simulink model "Microgrid"  (R2022b)
settings: Solver=ode45  StartTime=0.0  StopTime=0.5  RelTol=1e-3  EnableMultiTasking=on
undefined symbols (not defined in the file): AFPV, AFW, BMSS1, c1, c2, c3, c4, c5, c6, D1, Delta, DG, Ion, Lithium, pvc, R, wf1
libraries: spsDiodeLib x10, spsVoltageMeasurementLib x8, spsThreePhaseVIMeasurementLib x7, spsSeriesRLCBranchLib x7, fuzblock x6, sps_avr x5, spsMosfetLib x3, powerlib_extras x3, spsBreakerLib x2, spsThreePhaseParallelRLCLoadLib x2, spsThreePhaseBreakerLib x2, spsPWMGenerator2LevelLib x2
(part 1 of 2)
settings Model: Creator=Indhu  LastModifiedBy=zs
settings SolverCC: AlgebraicLoopSolver=TrustRegion
settings DataIOCC: LimitDataPoints=on  SaveFormat=Array  ReturnWorkspaceOutputs=off
settings OptimizationCC: LifeSpan=inf
settings DebuggingCC: SolverPrmCheckMsg=warning  UnconnectedInputMsg=warning  UnconnectedOutputMsg=warning  UnconnectedLineMsg=warning  SFUnexpectedBacktrackingDiag=warning  SFNoUnconditionalDefaultTransitionDiag=warning  SFExecutionAtInitializationDiag=none  SFMachineParentedDataDiag=warning  ArithmeticOperatorsInVariantConditions=warning
settings HardwareCC: ProdBitPerPointer=32  ProdBitPerSizeT=32  ProdBitPerPtrDiffT=32  ProdLargestAtomicFloat=None  ProdIntDivRoundTo=Undefined  ProdEndianess=Unspecified  ProdWordSize=32  ProdHWDeviceType=32-bit Generic
settings ModelReferenceCC: EnableRefExpFcnMdlSchedulingChecks=on  PropagateSignalLabelsOutOfModel=off
settings SFSimCC: SimUseLocalCustomCode=off  CustomCodeUndefinedFunction=UseInterfaceOnly
settings RTWCC: RTWUseLocalCustomCode=off
settings CodeAppCC: StateflowObjectComments=on
settings GRTTargetCC: TargetLangStandard=C89/C90 (ANSI)
settings ConfigComp: CovMetricSettings=dw  CovSaveCumulativeToWorkspaceVar=on  CovSaveSingleToWorkspaceVar=on  CovExternalEMLEnable=off  CovSFcnEnable=off
settings SimscapeCC: SimscapeNormalizeSystem=off

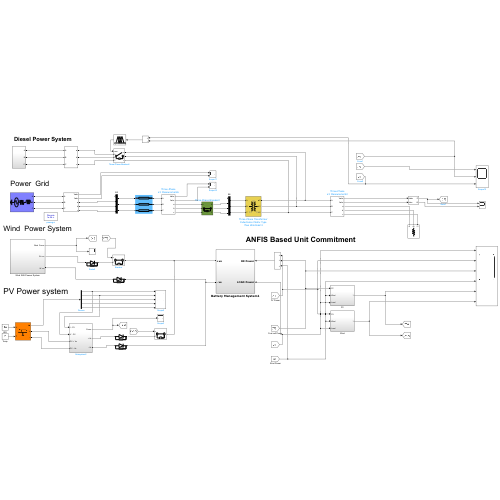
[thumbnail: Simulink's stored preview of the top-level diagram]
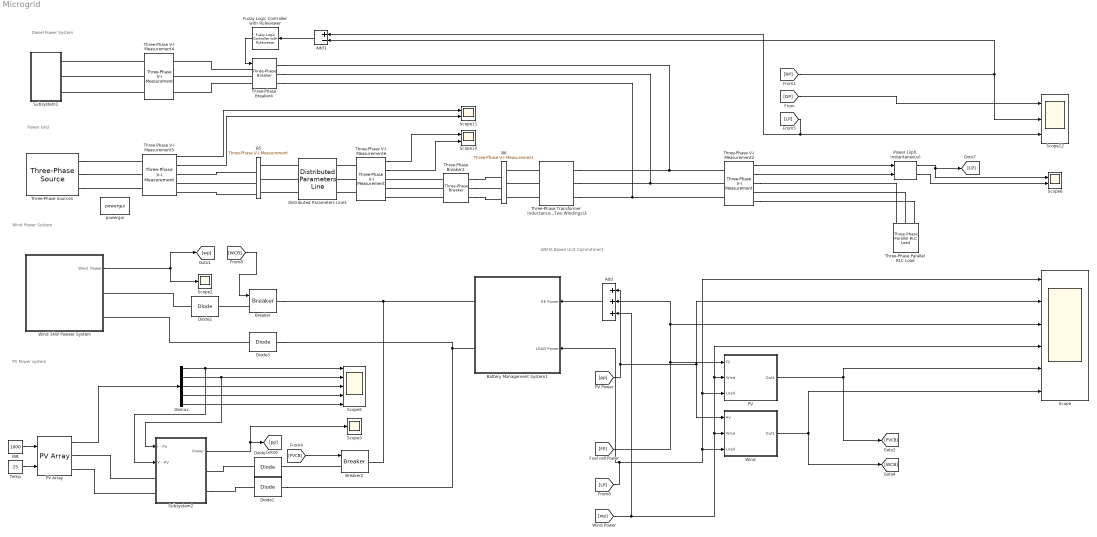
== system Microgrid ==
  note: ANFIS Based Unit Commitment
  note: Power Grid
  note: Wind Power System
  note: PV Power system
  note: Diesel Power System
  Add : Sum  Inputs=+++
  Add1 : Sum  Inputs=+-
  B5 : spsThreePhaseVIMeasurementLib/Three-Phase V-I Measurement  VoltageMeasurement=phase-to-ground  SetLabelV=off  LabelV=Vabc_B12  Vpu=off  VpuLL=off  CurrentMeasurement=no  SetLabelI=off  LabelI=A1  Ipu=off  Pbase=100e6  Vbase=25e3  OutputType=Magnitude  PhasorSimulation=off  PSBequivalent=0
  B6 : spsThreePhaseVIMeasurementLib/Three-Phase V-I Measurement  VoltageMeasurement=phase-to-phase  SetLabelV=off  LabelV=Vabc_B12  Vpu=off  VpuLL=off  CurrentMeasurement=no  SetLabelI=off  LabelI=A1  Ipu=off  Pbase=100e6  Vbase=440  OutputType=Magnitude  PhasorSimulation=off  PSBequivalent=0
  Battery Management System1 : Subsystem
  Breaker : spsBreakerLib/Breaker  InitialState=1  SwitchingTimes="[1/60  5/60]"  External=on  BreakerResistance=0.01  SnubberResistance=1e6  SnubberCapacitance=inf  Measurements=None  MoreParameters=on  NoBreakLoop=off
  Breaker2 : spsBreakerLib/Breaker  InitialState=1  SwitchingTimes="[1/60  5/60]"  External=on  BreakerResistance=0.01  SnubberResistance=1e6  SnubberCapacitance=inf  Measurements=None  MoreParameters=on  NoBreakLoop=off
  Demux : Demux  Outputs=5
  Diode{,1..3} (4 alike) : spsDiodeLib/Diode  Ron=0.001  Lon=0  Vf=0.8  IC=0  UseSnubber=off  Rs=500  Cs=250e-9  Measurements=off
  Distributed Parameters Line1 : spsDistributedParametersLineLib/Distributed Parameters Line  Phases=3  Length=100  Frequency=50  Resistance=[0.01273 0.3864]  Inductance="[0.9337e-3  4.1264e-3]"  Capacitance=[12.74e-9 7.751e-9]  x1=[-0.000566 2.76947894461141e-09 21710.1457186406 -60790.3871484274;-0.000565 2.76783586682722e-09 21729.2425103411 -60783.5637052244;-0.000564 2.76619251586859e-09 21748.3371574514 -60776.7342629242;-0.000563 2.7645488918977e-09 21767.4296580869 -60769.8988222007;-0.000562 2.76290499507677e-09 21786.5200103632 -60763.0573837288;-0.000561 2.76126082556805e-09 21805.6082123962 -60756.2099481834;-0.00056 2.75961638353382e-09 21824.6942623019 -60749.3565162406;-0.000559 2.75797166913637e-09 21843.7781581967 -60742.4970885766;-0.000558 2.75632668253802e-09 21862.859898197 -60735.6316658686;-0.000557 2.75468142390114e-09 21881.9394804195 -60728.760248794;-0.000556 2.7530358933881e-09 21901.0169029812 -60721.882838031;-0.000555 2.75139009116131e-09 21920.0921639991 -60714.9994342585;-0.000554 2.74974401738321e-09 21939.1652615907 -60708.1100381558;-0.000553 2.74809767221625e-09 21958.2361938735 -60701.2146504028;-0.000552 2.74645105582293e-09 21977.3049589653 -60694.3132716801;-0.000551 2.74480416836575e-09 21996.371554984 -60687.4059026689;-0.00055 2.74315701000726e-09 22015.4359800479 -60680.4925440508;-0.000549 2.74150958091003e-09 22034.4982322754 -60673.5731965082;-0.000548 2.73986188123666e-09 22053.5583097851 -60666.647860724;-0.000547 2.73821391114975e-09 22072.6162106958 -60659.7165373817;-0.000546 2.73656567081197e-09 22091.6719331267 -60652.7792271654;-0.000545 2.73491716038598e-09 22110.725475197 -60645.8359307598;-0.000544 2.73326838003449e-09 22129.7768350261 -60638.8866488502;-0.000543 2.73161932992023e-09 22148.8260107338 -60631.9313821223;-0.000542 2.72997001020595e-09 22167.8730004401 -60624.9701312628;-0.000541 2.72832042105443e-09 22186.9178022649 -60618.0028969586;-0.00054 2.72667056262848e-09 22205.9604143288 -60611.0296798973;-0.000539 2.72502043509093e-09 22225.0008347523 -60604.0504807672;-0.000538 2.72337003860465e-09 22244.0390616561 -60597.0653002572;-0.000537 2.72171937333252e-09 22263.0750931613 -60590.0741390566;-0.000536 2.72006843943746e-09 22282.108927389 -60583.0769978554;-0.000535 2.71841723708241e-09 22301.1405624608 -60576.0738773442;-0.000534 2.71676576643033e-09 22320.1699964982 -60569.0647782142;-0.000533 2.71511402764422e-09 22339.1972276232 -60562.0497011572;-0.000532 2.7134620208871e-09 22358.2222539578 -60555.0286468655;-0.000531 2.71180974632202e-09 22377.2450736243 -60548.0016160321;-0.00053 2.71015720411204e-09 22396.2656847453 -60540.9686093505;-0.000529 2.70850439442027e-09 22415.2840854435 -60533.9296275149;-0.000528 2.70685131740984e-09 22434.3002738418 -60526.8846712199;-0.000527 2.70519797324388e-09 22453.3142480635 -60519.8337411609;-0.000526 2.7035443620856e-09 22472.3260062319 -60512.7768380338;-0.000525 2.70189048409818e-09 22491.3355464706 -60505.713962535;-0.000524 2.70023633944486e-09 22510.3428669035 -60498.6451153617;-0.000523 2.6985819282889e-09 22529.3479656547 -60491.5702972114;-0.000522 2.69692725079358e-09 22548.3508408483 -60484.4895087826;-0.000521 2.69527230712221e-09 22567.3514906089 -60477.4027507739;-0.00052 2.69361709743813e-09 22586.3499130613 -60470.3100238849;-0.000519 2.69196162190471e-09 22605.3461063302 -60463.2113288156;-0.000518 2.69030588068532e-09 22624.340068541 -60456.1066662666;-0.000517 2.68864987394338e-09 22643.3317978189 -60448.996036939;-0.000516 2.68699360184234e-09 22662.3212922895 -60441.8794415347;-0.000515 2.68533706454567e-09 22681.3085500787 -60434.7568807561;-0.000514 2.68368026221685e-09 22700.2935693125 -60427.6283553061;-0.000513 2.68202319501941e-09 22719.2763481172 -60420.4938658883;-0.000512 2.68036586311689e-09 22738.2568846191 -60413.3534132068;-0.000511 2.67870826667286e-09 22757.2351769451 -60406.2069979663;-0.00051 2.67705040585093e-09 22776.211223222 -60399.0546208723;-0.000509 2.67539228081472e-09 22795.185021577 -60391.8962826305;-0.000508 2.67373389172787e-09 22814.1565701374 -60384.7319839476;-0.000507 2.67207523875407e-09 22833.1258670309 -60377.5617255305;-0.000506 2.67041632205702e-09 22852.0929103851 ...(+33023 chars)]  x2=[-0.000566 1.4266931735087e-08 21803.7450995725 -61159.0481551172;-0.000565 1.42603500349551e-08 21822.9577049232 -61152.1952886092;-0.000564 1.4253766927383e-08 21842.1681564344 -61145.3363866215;-0.000563 1.42471824130205e-08 21861.37645221 -61138.471449831;-0.000562 1.42405964925175e-08 21880.5825903542 -61131.6004789153;-0.000561 1.42340091665239e-08 21899.7865689715 -61124.7234745526;-0.00056 1.422742043569e-08 21918.9883861666 -61117.8404374214;-0.000559 1.4220830300666e-08 21938.1880400442 -61110.9513682013;-0.000558 1.42142387621023e-08 21957.3855287094 -61104.0562675721;-0.000557 1.42076458206495e-08 21976.5808502676 -61097.1551362142;-0.000556 1.42010514769582e-08 21995.7740028242 -61090.247974809;-0.000555 1.41944557316794e-08 22014.964984485 -61083.3347840379;-0.000554 1.41878585854639e-08 22034.1537933558 -61076.4155645834;-0.000553 1.4181260038963e-08 22053.3404275428 -61069.4903171284;-0.000552 1.41746600928277e-08 22072.5248851524 -61062.5590423563;-0.000551 1.41680587477097e-08 22091.7071642911 -61055.6217409513;-0.00055 1.41614560042602e-08 22110.8872630657 -61048.678413598;-0.000549 1.41548518631312e-08 22130.0651795833 -61041.7290609816;-0.000548 1.41482463249742e-08 22149.240911951 -61034.7736837882;-0.000547 1.41416393904413e-08 22168.4144582762 -61027.812282704;-0.000546 1.41350310601846e-08 22187.5858166666 -61020.8448584163;-0.000545 1.41284213348562e-08 22206.7549852301 -61013.8714116127;-0.000544 1.41218102151085e-08 22225.9219620748 -61006.8919429813;-0.000543 1.4115197701594e-08 22245.0867453089 -60999.9064532111;-0.000542 1.41085837949654e-08 22264.249333041 -60992.9149429915;-0.000541 1.41019684958754e-08 22283.4097233797 -60985.9174130126;-0.00054 1.40953518049769e-08 22302.5679144341 -60978.9138639649;-0.000539 1.4088733722923e-08 22321.7239043133 -60971.9042965397;-0.000538 1.40821142503667e-08 22340.8776911267 -60964.8887114288;-0.000537 1.40754933879615e-08 22360.0292729838 -60957.8671093246;-0.000536 1.40688711363609e-08 22379.1786479945 -60950.8394909201;-0.000535 1.40622474962183e-08 22398.3258142688 -60943.8058569089;-0.000534 1.40556224681875e-08 22417.470769917 -60936.7662079852;-0.000533 1.40489960529224e-08 22436.6135130496 -60929.7205448438;-0.000532 1.40423682510769e-08 22455.7540417771 -60922.6688681801;-0.000531 1.40357390633053e-08 22474.8923542106 -60915.61117869;-0.00053 1.40291084902618e-08 22494.0284484611 -60908.5474770702;-0.000529 1.40224765326008e-08 22513.1623226401 -60901.4777640177;-0.000528 1.40158431909768e-08 22532.293974859 -60894.4020402303;-0.000527 1.40092084660446e-08 22551.4234032296 -60887.3203064064;-0.000526 1.40025723584589e-08 22570.550605864 -60880.2325632449;-0.000525 1.39959348688747e-08 22589.6755808743 -60873.1388114453;-0.000524 1.39892959979472e-08 22608.798326373 -60866.0390517078;-0.000523 1.39826557463314e-08 22627.9188404728 -60858.933284733;-0.000522 1.39760141146829e-08 22647.0371212866 -60851.8215112224;-0.000521 1.39693711036571e-08 22666.1531669274 -60844.7037318778;-0.00052 1.39627267139096e-08 22685.2669755085 -60837.5799474016;-0.000519 1.39560809460963e-08 22704.3785451436 -60830.450158497;-0.000518 1.3949433800873e-08 22723.4878739464 -60823.3143658677;-0.000517 1.39427852788958e-08 22742.5949600308 -60816.172570218;-0.000516 1.39361353808208e-08 22761.699801511 -60809.0247722526;-0.000515 1.39294841073044e-08 22780.8023965016 -60801.8709726771;-0.000514 1.39228314590031e-08 22799.9027431171 -60794.7111721975;-0.000513 1.39161774365733e-08 22819.0008394724 -60787.5453715205;-0.000512 1.39095220406719e-08 22838.0966836827 -60780.3735713533;-0.000511 1.39028652719558e-08 22857.1902738631 -60773.1957724037;-0.00051 1.38962071310818e-08 22876.2816081293 -60766.0119753801;-0.000509 1.38895476187072e-08 22895.3706845971 -60758.8221809916;-0.000508 1.38828867354892e-08 22914.4575013823 -60751.6263899478;-0.000507 1.38762244820852e-08 22933.5420566012 -60744.4246029588;-0.000506 1.38695608591527e-08 22952.6243483703 -60737.2168207354 ...(+32976 chars)]  x3=[-0.000566 1.3679044311957e-10 55.3613635218509 -231.825545857438;-0.000565 1.36803348842223e-10 55.4341909318559 -231.808142132298;-0.000564 1.36816241062928e-10 55.5070128707255 -231.790715528612;-0.000563 1.3682911978041e-10 55.5798293312726 -231.773266048099;-0.000562 1.36841984993401e-10 55.6526403063105 -231.755793692482;-0.000561 1.36854836700628e-10 55.725445788653 -231.738298463486;-0.00056 1.36867674900825e-10 55.7982457711145 -231.720780362836;-0.000559 1.36880499592724e-10 55.8710402465099 -231.703239392262;-0.000558 1.36893310775059e-10 55.9438292076546 -231.685675553495;-0.000557 1.36906108446566e-10 56.0166126473649 -231.668088848268;-0.000556 1.36918892605982e-10 56.0893905584571 -231.650479278318;-0.000555 1.36931663252044e-10 56.1621629337484 -231.632846845383;-0.000554 1.36944420383494e-10 56.2349297660564 -231.615191551201;-0.000553 1.36957163999071e-10 56.3076910481993 -231.597513397517;-0.000552 1.36969894097518e-10 56.380446772996 -231.579812386075;-0.000551 1.36982610677578e-10 56.4531969332657 -231.562088518621;-0.00055 1.36995313737997e-10 56.5259415218281 -231.544341796906;-0.000549 1.3700800327752e-10 56.5986805315038 -231.52657222268;-0.000548 1.37020679294896e-10 56.6714139551137 -231.508779797697;-0.000547 1.37033341788872e-10 56.7441417854793 -231.490964523715;-0.000546 1.370459907582e-10 56.8168640154226 -231.473126402489;-0.000545 1.37058626201631e-10 56.8895806377663 -231.455265435783;-0.000544 1.37071248117918e-10 56.9622916453334 -231.437381625357;-0.000543 1.37083856505815e-10 57.0349970309477 -231.419474972977;-0.000542 1.37096451364077e-10 57.1076967874336 -231.401545480411;-0.000541 1.37109032691463e-10 57.1803909076157 -231.383593149428;-0.00054 1.37121600486729e-10 57.2530793843194 -231.3656179818;-0.000539 1.37134154748637e-10 57.3257622103708 -231.347619979301;-0.000538 1.37146695475945e-10 57.3984393785963 -231.329599143707;-0.000537 1.37159222667418e-10 57.4711108818229 -231.311555476797;-0.000536 1.37171736321817e-10 57.5437767128782 -231.293488980352;-0.000535 1.3718423643791e-10 57.6164368645905 -231.275399656155;-0.000534 1.37196723014461e-10 57.6890913297885 -231.257287505991;-0.000533 1.37209196050238e-10 57.7617401013014 -231.239152531647;-0.000532 1.3722165554401e-10 57.8343831719591 -231.220994734915;-0.000531 1.37234101494548e-10 57.9070205345921 -231.202814117584;-0.00053 1.37246533900623e-10 57.9796521820312 -231.184610681451;-0.000529 1.37258952761009e-10 58.0522781071081 -231.166384428312;-0.000528 1.37271358074479e-10 58.1248983026548 -231.148135359965;-0.000527 1.37283749839809e-10 58.1975127615041 -231.129863478212;-0.000526 1.37296128055776e-10 58.2701214764891 -231.111568784856;-0.000525 1.37308492721158e-10 58.3427244404437 -231.093251281702;-0.000524 1.37320843834736e-10 58.4153216462022 -231.074910970559;-0.000523 1.37333181395289e-10 58.4879130865996 -231.056547853237;-0.000522 1.37345505401601e-10 58.5604987544715 -231.038161931547;-0.000521 1.37357815852455e-10 58.6330786426538 -231.019753207306;-0.00052 1.37370112746637e-10 58.7056527439833 -231.001321682328;-0.000519 1.37382396082931e-10 58.7782210512971 -230.982867358434;-0.000518 1.37394665860127e-10 58.8507835574331 -230.964390237445;-0.000517 1.37406922077013e-10 58.9233402552296 -230.945890321185;-0.000516 1.37419164732379e-10 58.9958911375255 -230.927367611479;-0.000515 1.37431393825017e-10 59.0684361971605 -230.908822110156;-0.000514 1.37443609353721e-10 59.1409754269745 -230.890253819045;-0.000513 1.37455811317284e-10 59.2135088198082 -230.87166273998;-0.000512 1.37467999714503e-10 59.286036368503 -230.853048874796;-0.000511 1.37480174544174e-10 59.3585580659005 -230.834412225329;-0.00051 1.37492335805095e-10 59.4310739048432 -230.815752793419;-0.000509 1.37504483496068e-10 59.5035838781741 -230.797070580907;-0.000508 1.37516617615891e-10 59.5760879787366 -230.778365589638;-0.000507 1.37528738163369e-10 59.6485861993751 -230.759637821457;-0.000506 1.37540845137304e-10 59.7210785329341 ...(+33013 chars)]  x4=[-0.000566 -1.11527131730305e-10 80.4357788096744 -225.748148469716;-0.000565 -1.11550195139535e-10 80.506695711642 -225.722867684728;-0.000564 -1.11573247539202e-10 80.5776046679172 -225.697564621785;-0.000563 -1.11596288927031e-10 80.6485056715017 -225.672239283387;-0.000562 -1.11619319300748e-10 80.7193987153978 -225.646891672031;-0.000561 -1.1164233865808e-10 80.7902837926087 -225.62152179022;-0.00056 -1.11665346996754e-10 80.8611608961382 -225.596129640457;-0.000559 -1.11688344314501e-10 80.9320300189911 -225.570715225249;-0.000558 -1.1171133060905e-10 81.0028911541728 -225.545278547104;-0.000557 -1.11734305878133e-10 81.0737442946897 -225.519819608532;-0.000556 -1.11757270119482e-10 81.1445894335488 -225.494338412047;-0.000555 -1.1178022333083e-10 81.2154265637581 -225.468834960162;-0.000554 -1.11803165509913e-10 81.286255678326 -225.443309255396;-0.000553 -1.11826096654466e-10 81.3570767702622 -225.417761300267;-0.000552 -1.11849016762226e-10 81.4278898325768 -225.392191097297;-0.000551 -1.1187192583093e-10 81.4986948582809 -225.366598649009;-0.00055 -1.11894823858317e-10 81.5694918403863 -225.34098395793;-0.000549 -1.11917710842129e-10 81.6402807719056 -225.315347026588;-0.000548 -1.11940586780105e-10 81.7110616458522 -225.289687857512;-0.000547 -1.11963451669988e-10 81.7818344552403 -225.264006453235;-0.000546 -1.11986305509521e-10 81.8525991930849 -225.238302816293;-0.000545 -1.1200914829645e-10 81.9233558524019 -225.212576949221;-0.000544 -1.12031980028518e-10 81.9941044262079 -225.186828854559;-0.000543 -1.12054800703473e-10 82.0648449075201 -225.161058534848;-0.000542 -1.12077610319063e-10 82.1355772893569 -225.135265992631;-0.000541 -1.12100408873036e-10 82.2063015647372 -225.109451230454;-0.00054 -1.12123196363143e-10 82.2770177266808 -225.083614250866;-0.000539 -1.12145972787133e-10 82.3477257682083 -225.057755056415;-0.000538 -1.1216873814276e-10 82.4184256823411 -225.031873649654;-0.000537 -1.12191492427776e-10 82.4891174621014 -225.005970033138;-0.000536 -1.12214235639936e-10 82.5598011005122 -224.980044209423;-0.000535 -1.12236967776995e-10 82.6304765905974 -224.954096181067;-0.000534 -1.12259688836709e-10 82.7011439253814 -224.928125950633;-0.000533 -1.12282398816836e-10 82.7718030978897 -224.902133520682;-0.000532 -1.12305097715135e-10 82.8424541011486 -224.876118893781;-0.000531 -1.12327785529364e-10 82.9130969281851 -224.850082072496;-0.00053 -1.12350462257286e-10 82.983731572027 -224.824023059399;-0.000529 -1.12373127896662e-10 83.0543580257029 -224.797941857059;-0.000528 -1.12395782445254e-10 83.1249762822423 -224.771838468052;-0.000527 -1.12418425900828e-10 83.1955863346755 -224.745712894955;-0.000526 -1.12441058261148e-10 83.2661881760334 -224.719565140344;-0.000525 -1.1246367952398e-10 83.3367817993481 -224.693395206802;-0.000524 -1.12486289687092e-10 83.4073671976522 -224.667203096911;-0.000523 -1.12508888748253e-10 83.4779443639791 -224.640988813255;-0.000522 -1.12531476705231e-10 83.5485132913632 -224.614752358423;-0.000521 -1.12554053555798e-10 83.6190739728397 -224.588493735004;-0.00052 -1.12576619297725e-10 83.6896264014444 -224.562212945589;-0.000519 -1.12599173928785e-10 83.7601705702141 -224.535909992772;-0.000518 -1.12621717446752e-10 83.8307064721865 -224.509584879149;-0.000517 -1.12644249849401e-10 83.9012341003998 -224.483237607319;-0.000516 -1.12666771134509e-10 83.9717534478932 -224.456868179881;-0.000515 -1.12689281299852e-10 84.0422645077069 -224.430476599438;-0.000514 -1.12711780343209e-10 84.1127672728816 -224.404062868596;-0.000513 -1.12734268262359e-10 84.183261736459 -224.37762698996;-0.000512 -1.12756745055083e-10 84.2537478914815 -224.351168966141;-0.000511 -1.12779210719162e-10 84.3242257309926 -224.324688799748;-0.00051 -1.1280166525238e-10 84.3946952480361 -224.298186493397;-0.000509 -1.12824108652519e-10 84.4651564356572 -224.271662049702;-0.000508 -1.12846540917365e-10 84.5356092869016 -224.245115471281;-0.000507 -1.12868962044705e-10 84.6060537948158 -224.218546760755 ...(+33538 chars)]  x5=0.000565541566995743  V1=[0 0 0 2.339e-09 6.456e+04 6.456e+04;0 0 0 314.2 314.2 314.2;1.571 1.571 1.571 -0.9334 0.4129 -1.158]  V2=[0 0 0 9.955e-09 6.494e+04 6.494e+04;0 0 0 314.2 314.2 314.2;1.571 1.571 1.571 -1.047 0.4126 -1.158]  I1=[0 0 0 5.638e-11 239 239;0 0 0 314.2 314.2 314.2;1.571 1.571 1.571 -2.312 0.3045 -1.266]  I2=[0 0 0 5.238e-11 239.1 239.1;0 0 0 314.2 314.2 314.2;1.571 1.571 1.571 0.5382 0.4125 -1.158]  nHarmo=2  Measurements=None  Decoupling=off  VsMag0=0  VrMag0=0  VsAngle0=0  VrAngle0=0  IsMag0=0  IrMag0=0  IsAngle0=0  IrAngle0=0
      settings: LibrarySourceBlock=sps_lib/Power Grid Elements/Distributed Parameters Line
  Fuzzy Logic Controller with Ruleviewer : fuzblock/Fuzzy Logic  Controller  with Ruleviewer  fismatrix=[DG]  Ts=0.01
  IRR : Constant  Value=1000
  PV : Subsystem
  PV Array : spsPVArrayLib/PV Array  Npar=10  Nser=5  PlotType=array @ 25 deg.C & specified irradiances  S_vec="[ 1000  500  100 ]"  Temp_C_vec="[ 45 25  ]"  ModuleName=User-defined  PlotWhenSelected=off  Pm=334.905  Ncell=80  Voc=49.9  Isc=9  Vm=41.5  Im=8.07  beta_Voc_pc=-0.36  alpha_Isc_pc=0.09  beta_Voc=-0.17964  alpha_Isc=0.0081  IL=9.0297  I0=3.1312e-10  nI=1.0111  Rsh=77.6407  Rs=0.25633  RobustModel=off  RobustCellTemperature=313.3991  BAL=off  Tc=1e-6  Tfilter=5e-5
  "Power (3ph, Instantaneous)" : spsPower3phInstantaneousLib/Power (3ph, Instantaneous)
  Scope : Scope  NumInputPorts=6
  Scope10 : Scope  NumInputPorts=2
  Scope11 : Scope  NumInputPorts=2
  Scope12 : Scope  NumInputPorts=3
  Scope2 : Scope
  Scope3 : Scope
  Scope5 : Scope  NumInputPorts=5
  Scope6 : Scope  NumInputPorts=2
  Subsystem1 : Subsystem
  Subsystem2 : Subsystem
  "Temp " : Constant  Value=25
  Three-Phase Parallel RLC Load : spsThreePhaseParallelRLCLoadLib/Three-Phase Parallel RLC Load  LConnTagsString=A|B|C  Configuration=Delta  NominalVoltage=400  Vabc=[1e3 1e3 1e3]  Vabcp=[1e3 1e3 1e3]  NominalFrequency=50  UnbalancedPower=off  ActivePower=100e3  InductivePower=0  CapacitivePower=0  Pabc=[10e3 9e3 11e3]  QLabc=[100 90 110]  QCabc=[100 90 110]  Pabcp=[10e3 9e3 11e3]  QLabcp=[100 90 110]  QCabcp=[100 90 110]  Measurements=Branch voltages and currents  LoadType=constant PQ
  Three-Phase V-I Measurement2 : spsThreePhaseVIMeasurementLib/Three-Phase V-I Measurement  VoltageMeasurement=phase-to-phase  SetLabelV=off  LabelV=Vabc_b1  Vpu=off  VpuLL=off  CurrentMeasurement=yes  SetLabelI=off  LabelI=Iabc_b1  Ipu=off  Pbase=100e6  Vbase=500e3  OutputType=Complex  PhasorSimulation=off  PSBequivalent=0
  Three-Phase V-I Measurement4 : spsThreePhaseVIMeasurementLib/Three-Phase V-I Measurement  VoltageMeasurement=no  SetLabelV=off  LabelV=Vabc_b1  Vpu=off  VpuLL=off  CurrentMeasurement=no  SetLabelI=off  LabelI=Iabc_b1  Ipu=off  Pbase=100e6  Vbase=500e3  OutputType=Complex  PhasorSimulation=off  PSBequivalent=0
  Three-Phase V-I Measurement5 : spsThreePhaseVIMeasurementLib/Three-Phase V-I Measurement  VoltageMeasurement=phase-to-ground  SetLabelV=off  LabelV=Vabc  Vpu=off  VpuLL=off  CurrentMeasurement=yes  SetLabelI=off  LabelI=Iabc  Ipu=off  Pbase=100e6  Vbase=500e3  OutputType=Complex  PhasorSimulation=off  PSBequivalent=0
  Three-Phase V-I Measurement6 : spsThreePhaseVIMeasurementLib/Three-Phase V-I Measurement  VoltageMeasurement=phase-to-ground  SetLabelV=off  LabelV=Vabc  Vpu=off  VpuLL=off  CurrentMeasurement=yes  SetLabelI=off  LabelI=Iabc  Ipu=off  Pbase=100e6  Vbase=500e3  OutputType=Complex  PhasorSimulation=off  PSBequivalent=0
  Three-Phase Breaker2 : spsThreePhaseBreakerLib/Three-Phase Breaker  InitialState=closed  SwitchA=off  SwitchB=off  SwitchC=off  SwitchTimes="[1/50  20/50]"  External=off  BreakerResistance=0.001  SnubberResistance=1e6  SnubberCapacitance=inf  Measurements=None
  Three-Phase Breaker4 : spsThreePhaseBreakerLib/Three-Phase Breaker  InitialState=open  SwitchA=on  SwitchB=on  SwitchC=on  SwitchTimes=[0.02 1]  External=on  BreakerResistance=0.01  SnubberResistance=1e6  SnubberCapacitance=inf  Measurements=None
  Three-Phase Source1 : spsThreePhaseSourceLib/Three-Phase Source  InternalConnection=Yg  VoltagePhases=off  Voltage=63510.4  PhaseAngle=0  Voltage_phases=[25e3 25e3 25e3]/sqrt(3)  PhaseAngles_phases=[0 -120 +120]  Frequency=50  NonIdealSource=on  SpecifyImpedance=on  Resistance=0.8929  Inductance=16.58e-3  ShortCircuitLevel=100e6  BaseVoltage=63510.4  XRratio=7  BusType=swing  Pref=0  Qref=0  Prefabc=[10e3, 10e3, 10e3]  Qrefabc=[0, 0, 0]  Qmin=-inf  Qmax=inf
  Three-Phase Transformer Inductance Matrix Type (Two Windings)3 : spsThreePhaseTransformerInductanceMatrixTypeTwoWindingsLib/Three-Phase Transformer Inductance Matrix Type (Two Windings)  CoreType=Three-limb or five-limb core  Winding1Connection=Delta (D1)  Winding2Connection=Delta (D1)  AutoTransformer=off  Measurements=None  NominalPower=[100e3 50]  VLLnom=[63510.4 254.03]  WindingResistances=[0.01 0.01]  NoLoadIexcPos=2  NoLoadPlossPos=1000  ShortCircuitReactancePos=0.06  ShortCircuitReactancePosAuto=0.06  NoLoadIexcZero=100  NoLoadPlossZero=1500  ShortCircuitReactanceZero=0.03  ShortCircuitReactanceZeroAuto=0.03
      settings: LibrarySourceBlock=|
      | sps_lib/Power Grid Elements/Three-Phase Transformer
      | Inductance Matrix Type
      | (Two Windings)
  Wind : Subsystem
  Wind 3kW Poweer System : Subsystem
  powergui : spspowerguiLib/powergui  Priority=1  SimulationMode=Discrete  SampleTime=1e-6  frequency=60  Iterations=50  frequencyindice=0  Pbase=100e6  ErrMax=1e-4  UnitsV=kV  UnitsW=MW  buscounter=0  FunctionMessages=off  echomessages=off  EnableUseOfTLC=off  CurrentSourceSwitches=off  DisableSnubberDevices=off  DisableRonSwitches=off  DisableVfSwitches=off  DisplayEquations=off  AutomaticDiscreteSolvers=off  SolverType=Tustin  Interpol=off  ExternalGateDelay=off  methode=off  Ts=0  x0status=blocks  SPID=off  SwTol=0  HookPort=off  NonlinearTolerance=1e-4  nMaxIteration=100  ContinueOnMaxIteration=off  RestoreLinks=warning  ResistiveCurrentMeasurement=off  Frange=[0:2:500]  Ylog=off  Xlog=on  ShowGrid=off  save=off  variable=ZData  structure=ScopeData4  ZoomFFT=off  StartTime=0.1  cycles=3  DisplayStyle=1  fundamental=50  FreqAxis=off  MaxFrequency=1000  frequencyindicesteady=1  RmsSteady=1  display=off
  wires:
  Three-Phase V-I Measurement6/1 -> Scope10/1
  Three-Phase V-I Measurement6/2 -> Scope10/2
  Three-Phase V-I Measurement5/1 -> Scope11/1
  Three-Phase V-I Measurement5/2 -> Scope11/2
  Demux/5 -> Scope5/5
  Demux/4 -> Scope5/4
  Demux/1 -> Subsystem2/2(V - PV), Scope5/1
  Demux/3 -> Scope5/3
  Demux/2 -> Subsystem2/1(I - PV), Scope5/2
  PV Array/1 -> Demux/1
  "Temp "/1 -> PV Array/2
  IRR/1 -> PV Array/1
  Subsystem2/1(Power) -> Scope3/1, [pp]
  Wind 3kW Poweer System/1(Wind  Power) -> Scope2/1, [wp]
  Three-Phase V-I Measurement2/1 -> "Power (3ph, Instantaneous)"/1
  Three-Phase V-I Measurement2/2 -> "Power (3ph, Instantaneous)"/2
  [PVCB] -> Breaker2/1
  [WCB] -> Breaker/1
  PV/1(Out1) -> [PVCB], Scope/5
  [LP] -> Battery Management System1/2(LOAD Power), Wind/3(Load), PV/3(Load), Scope/1
  [pp] -> Wind/1(PV), Scope/2, Add/1
  [wp] -> Scope/4, PV/2(Wind), Wind/2(Wind), Add/3
  Wind/1(Out1) -> [WCB], Scope/6
  [FP] -> PV/1(FC), Add/2, Scope/3
  Add/1 -> Battery Management System1/1(RE Power)
  "Power (3ph, Instantaneous)"/2 -> Scope6/2
  "Power (3ph, Instantaneous)"/1 -> [LP], Scope6/1
  [DP] -> Scope12/1
  [RP] -> Scope12/2, Add1/2
  [LP] -> Add1/1, Scope12/3
  Add1/1 -> Fuzzy Logic Controller with Ruleviewer/1
  Fuzzy Logic Controller with Ruleviewer/1 -> Three-Phase Breaker4/1
  connections:
  Three-Phase Breaker2/LConn3 -- B6/RConn3
  Three-Phase V-I Measurement6/LConn1 -- Distributed Parameters Line1/RConn1
  Three-Phase Transformer Inductance Matrix Type (Two Windings)3/LConn1 -- B6/LConn1
  B5/RConn1 -- Three-Phase V-I Measurement5/RConn1
  Three-Phase Source1/RConn3 -- Three-Phase V-I Measurement5/LConn3
  Three-Phase Breaker2/RConn1 -- Three-Phase V-I Measurement6/RConn1
  Three-Phase Source1/RConn1 -- Three-Phase V-I Measurement5/LConn1
  Three-Phase V-I Measurement6/LConn2 -- Distributed Parameters Line1/RConn2
  Three-Phase Transformer Inductance Matrix Type (Two Windings)3/LConn3 -- B6/LConn3
  Three-Phase Breaker2/LConn1 -- B6/RConn1
  Three-Phase Breaker2/LConn2 -- B6/RConn2
  Three-Phase Breaker2/RConn2 -- Three-Phase V-I Measurement6/RConn2
  Three-Phase V-I Measurement6/LConn3 -- Distributed Parameters Line1/RConn3
  Three-Phase Transformer Inductance Matrix Type (Two Windings)3/LConn2 -- B6/LConn2
  Distributed Parameters Line1/LConn1 -- B5/LConn1
  B5/RConn2 -- Three-Phase V-I Measurement5/RConn2
  Distributed Parameters Line1/LConn2 -- B5/LConn2
  Distributed Parameters Line1/LConn3 -- B5/LConn3
  B5/RConn3 -- Three-Phase V-I Measurement5/RConn3
  Three-Phase Breaker2/RConn3 -- Three-Phase V-I Measurement6/RConn3
  Three-Phase Source1/RConn2 -- Three-Phase V-I Measurement5/LConn2
  Three-Phase Breaker4/RConn1 -- Three-Phase V-I Measurement2/LConn1 -- Three-Phase Transformer Inductance Matrix Type (Two Windings)3/RConn1
  Three-Phase Breaker4/RConn3 -- Three-Phase V-I Measurement2/LConn3 -- Three-Phase Transformer Inductance Matrix Type (Two Windings)3/RConn3
  Three-Phase Breaker4/RConn2 -- Three-Phase V-I Measurement2/LConn2 -- Three-Phase Transformer Inductance Matrix Type (Two Windings)3/RConn2
  Diode/LConn1 -- Subsystem2/RConn1
  Subsystem2/RConn2 -- Diode1/LConn1
  PV Array/RConn1 -- Subsystem2/LConn1
  PV Array/RConn2 -- Subsystem2/LConn2
  Battery Management System1/RConn1 -- Breaker2/RConn1 -- Breaker/RConn1
  Diode1/RConn1 -- Diode3/RConn1 -- Battery Management System1/RConn2
  Diode2/LConn1 -- Wind 3kW Poweer System/RConn1
  Diode3/LConn1 -- Wind 3kW Poweer System/RConn2
  Breaker/LConn1 -- Diode2/RConn1
  Breaker2/LConn1 -- Diode/RConn1
  Three-Phase V-I Measurement2/RConn1 -- Three-Phase Parallel RLC Load/LConn1
  Three-Phase Parallel RLC Load/LConn2 -- Three-Phase V-I Measurement2/RConn2
  Three-Phase V-I Measurement2/RConn3 -- Three-Phase Parallel RLC Load/LConn3
  Three-Phase V-I Measurement4/LConn1 -- Subsystem1/RConn1
  Three-Phase Breaker4/LConn2 -- Three-Phase V-I Measurement4/RConn2
  Three-Phase Breaker4/LConn1 -- Three-Phase V-I Measurement4/RConn1
  Three-Phase V-I Measurement4/LConn3 -- Subsystem1/RConn3
  Three-Phase Breaker4/LConn3 -- Three-Phase V-I Measurement4/RConn3
  Three-Phase V-I Measurement4/LConn2 -- Subsystem1/RConn2
